simulink model "Sfuntion_sim"  (R2020b)
settings: Solver=VariableStepAuto  StartTime=0.0  StopTime=50  RelTol=1e-3
libraries: simulink x1
settings Model: Creator=zhiyao  LastModifiedBy=zhiyao

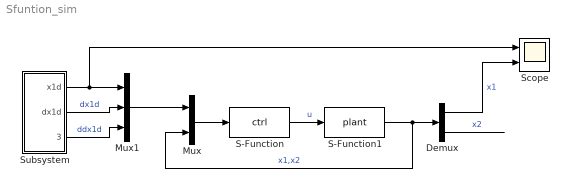
== system Sfuntion_sim ==
  Demux : Demux  Outputs=2
  Mux : Mux  Inputs=2
  Mux1 : Mux  Inputs=3
  S-Function : S-Function  FunctionName=ctrl  Parameters=pa  SFunctionDeploymentMode=off  EnableBusSupport=off
  S-Function1 : S-Function  FunctionName=plant  Parameters=pa  SFunctionDeploymentMode=off  EnableBusSupport=off
  Scope : Scope  NumInputPorts=2
  Subsystem : Subsystem
  wires:
  S-Function/1 -> S-Function1/1  "u"
  S-Function1/1 -> Mux/2, Demux/1  "x1,x2"
  Demux/1 -> Scope/2  "x1"
  Demux/2 -> ?  "x2"
  Subsystem/1(x1d) -> Mux1/1, Scope/1
  Subsystem/2(dx1d) -> Mux1/2  "dx1d"
  Subsystem/3(ddx1d) -> Mux1/3  "ddx1d"
  Mux1/1 -> Mux/1
  Mux/1 -> S-Function/1

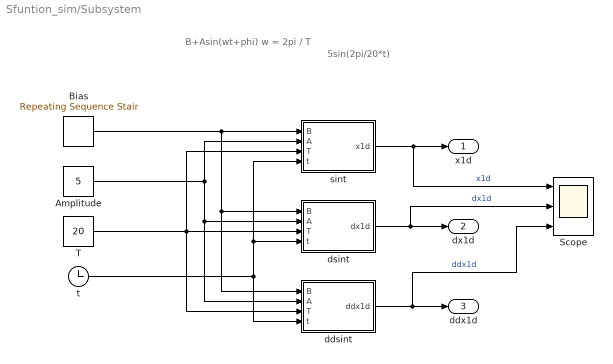
== system Sfuntion_sim/Subsystem ==
  note: 5sin(2pi/20*t)
  note: B+Asin(wt+phi)
      | w = 2pi / T
  Amplitude : Constant  Value=5
  Bias : simulink/Sources/Repeating Sequence Stair  OutValues=[0,1,2,3,4].'  tsamp=10  OutMin=[]  OutMax=[]  OutDataTypeStr=double  OutputDataTypeScalingMode=double  OutDataType=fixdt(0,8)  ConRadixGroup=Best Precision: Vector-wise  OutScaling=2^-12
  Scope : Scope  NumInputPorts=3
  T : Constant  Value=20
  ddsint : MATLAB Function  TreatAsAtomicUnit=on
  dsint : MATLAB Function  TreatAsAtomicUnit=on
  sint : MATLAB Function  TreatAsAtomicUnit=on
  t : Clock
  x1d : Outport
  dx1d : Outport  Port=2
  ddx1d : Outport  Port=3
  wires:
  Bias/1 -> ddsint/1(B), dsint/1(B), sint/1(B)
  t/1 -> ddsint/4(t), dsint/4(t), sint/4(t)
  Amplitude/1 -> ddsint/2(A), dsint/2(A), sint/2(A)
  T/1 -> sint/3(T), ddsint/3(T), dsint/3(T)
  sint/1(x1d) -> Scope/1, x1d/1  "x1d"
  ddsint/1(ddx1d) -> Scope/3, ddx1d/1  "ddx1d"
  dsint/1(dx1d) -> Scope/2, dx1d/1  "dx1d"

== matlab function Sfuntion_sim/Subsystem/sint ==
  data: B input; x1d output; A input; T input; t input
function x1d = fc(B,A,T,t)

x1d = B+A*sin(2*pi/T*t);

== matlab function Sfuntion_sim/Subsystem/dsint ==
  data: B input; dx1d output; A input; T input; t input
function dx1d = fc(B,A,T,t)

dx1d = A*2*pi/T*cos(2*pi/T*t);

== matlab function Sfuntion_sim/Subsystem/ddsint ==
  data: B input; ddx1d output; A input; T input; t input
function ddx1d = fc(B,A,T,t)

ddx1d = -2*pi/T*A*2*pi/T*sin(2*pi/T*t);
